simulink model "controller_only_masterslave"  (R2016a)
settings: Solver=FixedStepAuto  StartTime=0.0  StopTime=25  FixedStep=0.1  RelTol=1e-3
settings Model: ExtModeTrigDuration=5  Creator=aless  LastModifiedBy=aless
settings OptimizationCC: DefaultParameterBehavior=Inlined  OptimizeModelRefInitCode=on  LifeSpan=1
settings HardwareCC: ProdBitPerPointer=32  ProdLargestAtomicInteger=Long  ProdLargestAtomicFloat=Double  ProdWordSize=32  ProdHWDeviceType=ARM Compatible->ARM Cortex
settings RTWCC: SystemTargetFile=ert.tlc  GenCodeOnly=on  TemplateMakefile=ert_default_tmf  GenerateReport=on  IncludeHyperlinkInReport=on  LaunchReport=on  GenerateTraceInfo=on  GenerateTraceReport=on  GenerateTraceReportSl=on  GenerateTraceReportSf=on  GenerateTraceReportEml=on
settings CodeAppCC: ForceParamTrailComments=on  OperatorAnnotations=on  SimulinkDataObjDesc=on  SFDataObjDesc=on  MATLABFcnDesc=on  InsertBlockDesc=on  MATLABSourceComments=on
settings ERTTargetCC: GenerateSampleERTMain=on  MultiInstanceERTCode=on  CodeInterfacePackaging=Reusable function  InlinedParameterPlacement=NonHierarchical  RootIOFormat=Structure reference  ERTCustomFileTemplate=example_file_process.tlc  ERTFilePackagingFormat=Compact

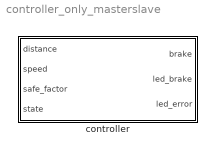
== system controller_only_masterslave ==
  controller : Subsystem

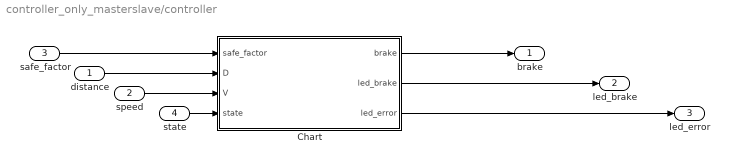
== system controller_only_masterslave/controller ==
  distance : Inport
  speed : Inport  Port=2
  safe_factor : Inport  Port=3
  state : Inport  Port=4
  Chart : Stateflow chart  TreatAsAtomicUnit=on
  brake : Outport
  led_brake : Outport  Port=2
  led_error : Outport  Port=3
  wires:
  distance/1 -> Chart/2(D)
  speed/1 -> Chart/3(V)
  safe_factor/1 -> Chart/1(safe_factor)
  Chart/1(brake) -> brake/1
  state/1 -> Chart/4(state)
  Chart/2(led_brake) -> led_brake/1
  Chart/3(led_error) -> led_error/1

== stateflow chart controller_only_masterslave/controller/Chart ==
  state INIT_STATE
    en: brake = uint8(0),
    led_brake = uint8(0),
    led_error = uint8(0);
  state UNSAFE_DISTANCE
    en: brake = uint8(1);
    state LED_ON
      en: led_brake = uint8(1);
    state LED_OFF
      en: led_brake = uint8(0);
    (default) -> LED_ON
    LED_OFF -> LED_ON : after(1/(1+V^2/100-D), msec)
    LED_ON -> LED_OFF : after(1/(1+V^2/100-D), msec)
  state SAFE_DISTANCE
    en: brake = uint8(0),
    led_brake = uint8(0);
  state MALFUNCTION
    en: brake = uint8(0),
    led_brake = uint8(0),
    led_error = uint8(1);
  (default) -> INIT_STATE
  INIT_STATE -> UNSAFE_DISTANCE [order 2] : [(D <= (V^2)/100) && state ~= 1]
  INIT_STATE -> SAFE_DISTANCE [order 1] : [(D > (V^2)/100) && state ~= 1]
  INIT_STATE -> MALFUNCTION [order 3] : [state == 1]
  SAFE_DISTANCE -> UNSAFE_DISTANCE [order 1] : [(D <= (V^2)/100) && state ~= 1]
  UNSAFE_DISTANCE -> SAFE_DISTANCE [order 1] : [(D > (V^2)/100 * safe_factor) && state ~= 1]
  SAFE_DISTANCE -> MALFUNCTION [order 2] : [state == 1]
  UNSAFE_DISTANCE -> MALFUNCTION [order 2] : [state == 1]
  MALFUNCTION -> MALFUNCTION
  data: safe_factor input; brake output; D input; V input; state input; led_brake output; led_error output
